simulink model "SIM_nonlinear_LQR_dis"  (R2016a)
settings: Solver=ode23t  SolverMode=SingleTasking  StartTime=0.0  StopTime=30  MaxStep=1e-4  RelTol=1e-3
undefined symbols (not defined in the file): input_dis, input_dis_time, K, Kr
libraries: dspsrcs4 x3
settings Model: Creator=edzel  LastModifiedBy=edzel
settings DataIOCC: ReturnWorkspaceOutputs=on
settings DebuggingCC: UnconnectedInputMsg=none  UnconnectedOutputMsg=none  UnconnectedLineMsg=none  SFUnexpectedBacktrackingDiag=error  SFNoUnconditionalDefaultTransitionDiag=error
settings ModelReferenceCC: EnableRefExpFcnMdlSchedulingChecks=off
settings SFSimCC: SimUseLocalCustomCode=on
settings RTWCC: Description=Generic Real-Time Target  RTWUseLocalCustomCode=on
settings GRTTargetCC: TargetLangStandard=C99 (ISO)
settings ConfigComp: CovMetricSettings=dwe  CovSaveCumulativeToWorkspaceVar=off  CovSaveSingleToWorkspaceVar=off  CovExternalEMLEnable=on

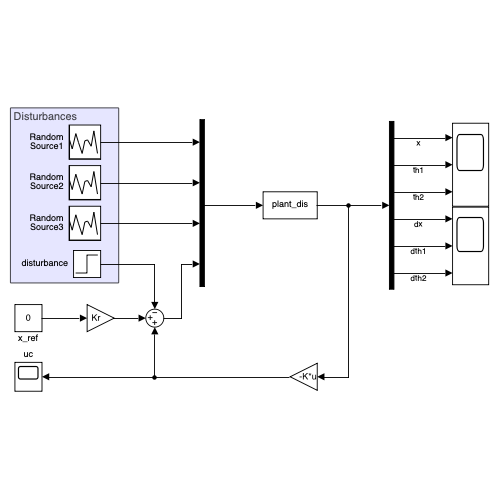
[thumbnail: Simulink's stored preview of the top-level diagram]
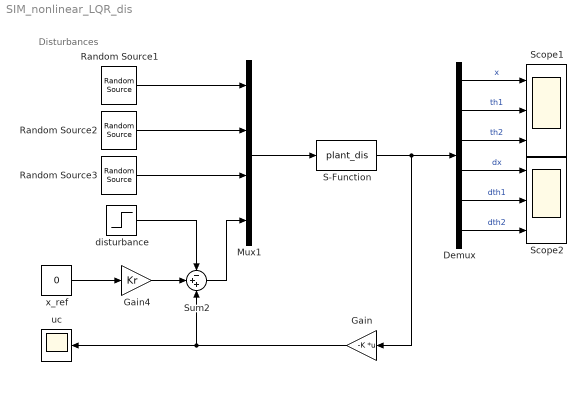
== system SIM_nonlinear_LQR_dis ==
  note: Disturbances
  Demux : Demux  Outputs=6
  Gain : Gain  Gain=-K  Multiplication=Matrix(K*u)
  Gain4 : Gain  Gain=Kr
  Mux1 : Mux
  Random Source1 : dspsrcs4/Random Source  SrcType=Gaussian  NormMethod=Ziggurat  CltLength=12  MinVal=0  MaxVal=1  MeanVal=d1_mean  VarVal=d1_variance  RepMode=Specify seed  rawSeed=42  IsInherit=off  SampMode=Continuous  SampTime=1  SampFrame=1  DataType=Double  OutComplex=Real  OutputFrames=off
  Random Source2 : dspsrcs4/Random Source  SrcType=Gaussian  NormMethod=Ziggurat  CltLength=12  MinVal=0  MaxVal=1  MeanVal=d2_mean  VarVal=d2_variance  RepMode=Specify seed  rawSeed=42  IsInherit=off  SampMode=Continuous  SampTime=1  SampFrame=1  DataType=Double  OutComplex=Real  OutputFrames=off
  Random Source3 : dspsrcs4/Random Source  SrcType=Gaussian  NormMethod=Ziggurat  CltLength=12  MinVal=0  MaxVal=1  MeanVal=d3_mean  VarVal=d3_variance  RepMode=Specify seed  rawSeed=42  IsInherit=off  SampMode=Continuous  SampTime=1  SampFrame=1  DataType=Double  OutComplex=Real  OutputFrames=off
  S-Function : S-Function  FunctionName=plant_dis  Parameters=CoeF1, CoeF2, CoeF3, theta1_rad, theta2_rad  SFunctionDeploymentMode=off  EnableBusSupport=off
  Scope1 : Scope  NumInputPorts=3
  Scope2 : Scope  NumInputPorts=3
  Sum2 : Sum  Inputs=-++
  disturbance : Step  Time=input_dis_time  After=input_dis  SampleTime=0
  uc : Scope
  x_ref : Constant  Value=0
  wires:
  x_ref/1 -> Gain4/1
  Gain4/1 -> Sum2/2
  Gain/1 -> Sum2/3, uc/1
  disturbance/1 -> Sum2/1
  Random Source3/1 -> Mux1/3
  Random Source2/1 -> Mux1/2
  Random Source1/1 -> Mux1/1
  Mux1/1 -> S-Function/1
  Sum2/1 -> Mux1/4
  S-Function/1 -> Demux/1, Gain/1
  Demux/4 -> Scope2/1  "dx"
  Demux/3 -> Scope1/3  "th2"
  Demux/5 -> Scope2/2  "dth1"
  Demux/6 -> Scope2/3  "dth2"
  Demux/2 -> Scope1/2  "th1"
  Demux/1 -> Scope1/1  "x"
